simulink model "Sim34"  (R2019a)
settings: Solver=VariableStepAuto  StartTime=0.0  StopTime=10.0  RelTol=1e-3
settings Model: Creator=fbleo  LastModifiedBy=fbleo

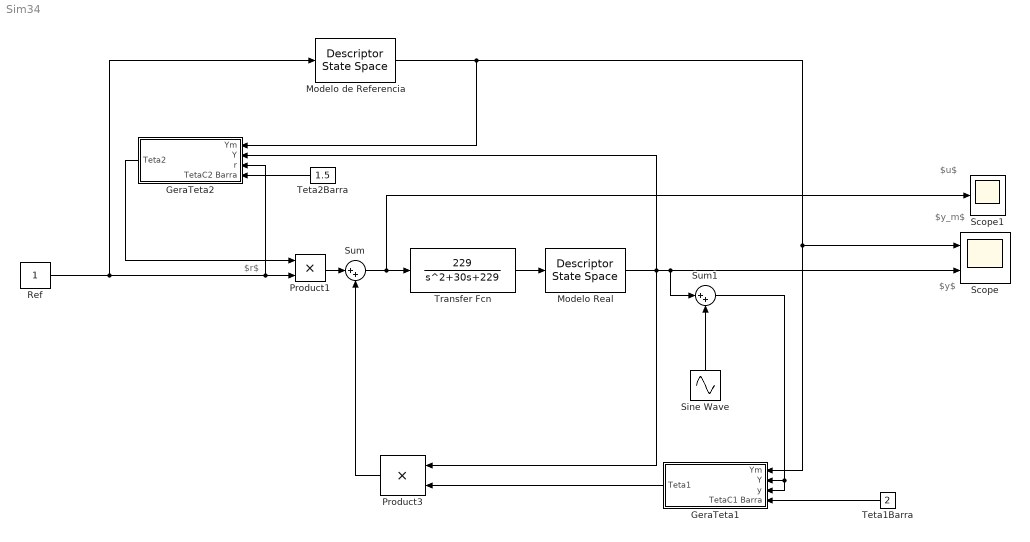
== system Sim34 ==
  note: $u$
  note: $y$
  note: $y_m$
  note: $r$
  GeraTeta1 : Subsystem
  GeraTeta2 : Subsystem
  Modelo Real : DescriptorStateSpace  A=-1  B=2  D=0  InitialCondition=0.5
  Modelo de Referencia : DescriptorStateSpace  A=-3  B=3  D=0  InitialCondition=0
  Product1 : Product
  Product3 : Product
  Ref : Constant
  Scope : Scope  NumInputPorts=2
  Scope1 : Scope
  Sine Wave : Sin  Amplitude=0.1  Frequency=16.1  SampleTime=0
  Sum : Sum  Inputs=|++
  Sum1 : Sum  Inputs=|++
  Teta1Barra : Constant  Value=2
  Teta2Barra : Constant  Value=1.5
  Transfer Fcn : TransferFcn  Numerator=[229]  Denominator=[1 30 229]
  wires:
  Product1/1 -> Sum/1
  GeraTeta2/1(Teta2) -> Product1/1
  Teta2Barra/1 -> GeraTeta2/4(TetaC2 Barra)
  Product3/1 -> Sum/2
  Ref/1 -> Modelo de Referencia/1, Product1/2, GeraTeta2/3(r)
  Sum/1 -> Transfer Fcn/1, Scope1/1
  Teta1Barra/1 -> GeraTeta1/4(TetaC1 Barra)
  Transfer Fcn/1 -> Modelo Real/1
  Modelo Real/1 -> Scope/2, Sum1/1, Product3/1, GeraTeta2/2(Y)
  Modelo de Referencia/1 -> GeraTeta1/1(Ym), Scope/1, GeraTeta2/1(Ym)
  GeraTeta1/1(Teta1) -> Product3/2
  Sum1/1 -> GeraTeta1/3(y), GeraTeta1/2(Y)
  Sine Wave/1 -> Sum1/2

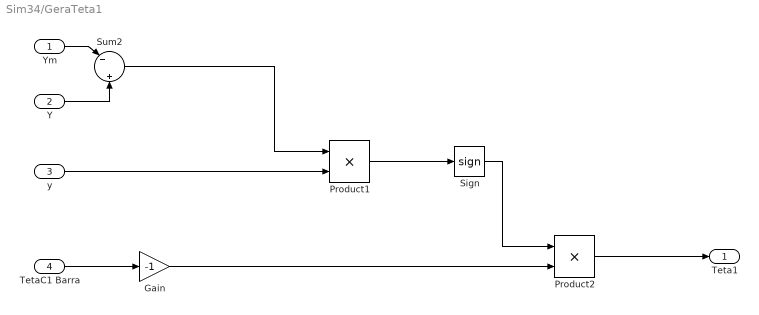
== system Sim34/GeraTeta1 ==
  Ym : Inport
  Y : Inport  Port=2
  y : Inport  Port=3
  TetaC1 Barra : Inport  Port=4
  Gain : Gain  Gain=-1
  Product1 : Product
  Product2 : Product
  Sign : Signum
  Sum2 : Sum  Inputs=|-||+
  Teta1 : Outport
  wires:
  y/1 -> Product1/2
  TetaC1 Barra/1 -> Gain/1
  Product2/1 -> Teta1/1
  Ym/1 -> Sum2/1
  Sign/1 -> Product2/1
  Y/1 -> Sum2/2
  Sum2/1 -> Product1/1
  Gain/1 -> Product2/2
  Product1/1 -> Sign/1

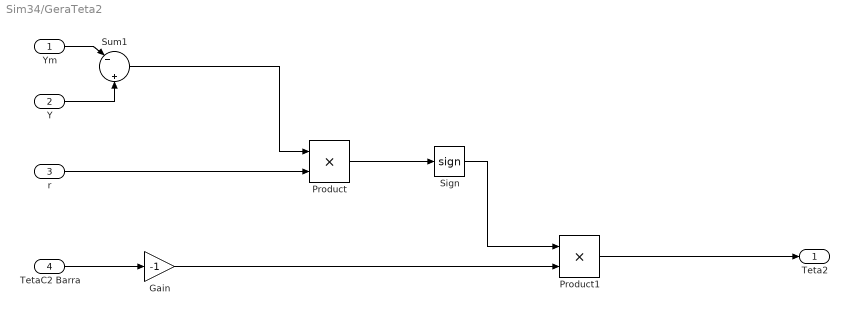
== system Sim34/GeraTeta2 ==
  Ym : Inport
  Y : Inport  Port=2
  r : Inport  Port=3
  TetaC2 Barra : Inport  Port=4
  Gain : Gain  Gain=-1
  Product : Product
  Product1 : Product
  Sign : Signum
  Sum1 : Sum  Inputs=|-||+
  Teta2 : Outport
  wires:
  Ym/1 -> Sum1/1
  Y/1 -> Sum1/2
  Sum1/1 -> Product/1
  r/1 -> Product/2
  TetaC2 Barra/1 -> Gain/1
  Gain/1 -> Product1/2
  Product1/1 -> Teta2/1
  Product/1 -> Sign/1
  Sign/1 -> Product1/1
